simulink model "pro6"  (R2020a)
settings: Solver=VariableStepAuto  StartTime=0.0  StopTime=10.0  RelTol=1e-3
undefined symbols (not defined in the file): A, B, C, D
settings Model: Creator=007  LastModifiedBy=007

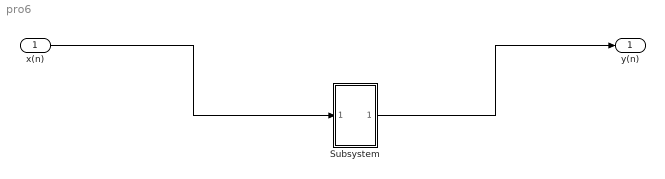
== system pro6 ==
  x(n) : Inport
  Subsystem : Subsystem
  y(n) : Outport
  wires:
  x(n)/1 -> Subsystem/1(In1)
  Subsystem/1(Out1) -> y(n)/1

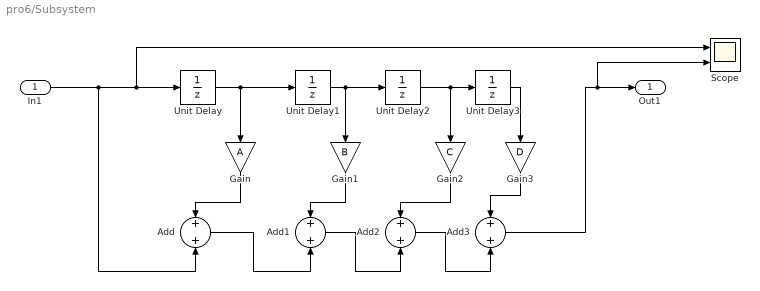
== system pro6/Subsystem ==
  In1 : Inport
  Add{,1..3} (4 alike) : Sum
  Gain : Gain  Gain=A
  Gain1 : Gain  Gain=B
  Gain2 : Gain  Gain=C
  Gain3 : Gain  Gain=D
  Scope : Scope  NumInputPorts=2
  Unit Delay{,1..3} (4 alike) : UnitDelay  SampleTime=-1  HasFrameUpgradeWarning=on
  Out1 : Outport
  wires:
  In1/1 -> Add/2, Scope/1, Unit Delay/1
  Unit Delay/1 -> Gain/1, Unit Delay1/1
  Unit Delay1/1 -> Unit Delay2/1, Gain1/1
  Add1/1 -> Add2/2
  Gain3/1 -> Add3/1
  Gain/1 -> Add/1
  Unit Delay3/1 -> Gain3/1
  Gain1/1 -> Add1/1
  Unit Delay2/1 -> Gain2/1, Unit Delay3/1
  Gain2/1 -> Add2/1
  Add/1 -> Add1/2
  Add2/1 -> Add3/2
  Add3/1 -> Scope/2, Out1/1
